simulink model "GFOL_nonlinear"  (R2020a)
settings: Solver=ode3  StartTime=0.0  StopTime=Tsim  FixedStep=T_solver  RelTol=1e-6
values from neighbouring files (symbols this model uses):
  f_n1 = f1    (= 50)    [param.m]
  Ipeak_n1 = Sn_n1*sqrt(2)/(sqrt(3)*Un_n1)    [linearization_point.m]    (also in param.m = Sn_n1/(sqrt(3)*Un_n1))
  k_droop_f_n1 = 20*Sn_n1/w_n1    (= 175070.437401)    [param.m]
  k_droop_u_n1 = 0.3*50*Sn_n1/Vpeak_n1    [param.m]
  ki_P_n1 = 1e-3*1/tau_p    (= 0.01)    [param.m]
  ki_pll_n1 = kp_pll_n1/tau_pll_n1    [param.m]
  ki_Q_n1 = 1e-3*1/tau_q    (= 0.01)    [param.m]
  ki_s_n1 = Rc_n1/taus    (= 0.865636363636)    [param.m]
  kp_P_n1 = 1e-3*taus/tau_p    (= 1e-05)    [param.m]
  kp_pll_n1 = xi_pll_n1*2*omega_pll_n1/Vpeak_n1    [param.m]
  kp_Q_n1 = 1e-3*taus/tau_q    (= 1e-05)    [param.m]
  kp_s_n1 = Lc_n1/taus    (= 0.0826621837157)    [param.m]
  Lc_n1 = 0.15*Ln_n1    (= 8.26621837157e-05)    [param.m]
  Lg_n1 = Xg_n1/w_g1    [param.m]
  Lg_n2 = imag(Zg_n2)/w_g1    [param.m]
  P_ref_n1 = 0.5*Sn_n1    (= 1375000)    [param.m]
  plots_step = 10e-6    (= 1e-05)    [param.m]
  Q_ref_n1 = 0.1*Sn_n1    (= 275000)    [param.m]
  Rc_n1 = 0.005*Xn_n1    (= 0.000865636363636)    [param.m]
  Rg_n1 = sqrt(Xcc1^2/(XR_ratio^2+1))    [param.m]
  Rg_n2 = real(Zg_n2)    [param.m]
  Sn_n1 = Sn1    (= 2750000)    [param.m]
  T_solver = 10e-6    (= 1e-05)    [param.m]
  T_step = 2    [param.m]
  tau_droop_f = 1/50    (= 0.02)    [param.m]
  tau_droop_u = 1/50    (= 0.02)    [param.m]
  Vdcref_n1 = 2e3    (= 2000)    [param.m]
  Vpeak_g1_fnl = Vpeak_n1*0.98    [param.m]
  Vpeak_n1 = Un_n1/sqrt(3)*sqrt(2)    [param.m]
  Vpeak_q1_init = Vpeak_n1*1    [param.m]
  w_n1 = 2*pi*f_n1    (= 314.159265359)    [param.m]
undefined symbols (not defined in the file or in its folder): P_set, P_step, Q_set, Q_step, t_ramp, t_step_P, t_step_Q, tau_ramp
libraries: powerlib x37, simulink x5, simulink_extras x1
(part 1 of 2)
settings Model: SimulationMode=accelerator  ExtModeTrigDuration=100  Creator=Enric  LastModifiedBy=Saman
settings SolverCC: SolverJacobianMethodControl=FullPerturbation  AutoInsertRateTranBlk=on
settings DataIOCC: LimitDataPoints=on  SaveOutput=off  ReturnWorkspaceOutputs=off  StateSaveName=tmp_raccel_xout  SignalLoggingName=tmp_raccel_logsout
settings OptimizationCC: EfficientMapNaN2IntZero=off  LifeSpan=inf
settings DebuggingCC: AllowSymbolicDim=off  SFUnexpectedBacktrackingDiag=warning  SFNoUnconditionalDefaultTransitionDiag=warning  SFExecutionAtInitializationDiag=none  ArithmeticOperatorsInVariantConditions=warning
settings HardwareCC: TargetBitPerPointer=64  TargetBitPerSizeT=64  TargetBitPerPtrDiffT=64  TargetLongLongMode=on  TargetIntDivRoundTo=Zero  TargetEndianess=LittleEndian  TargetWordSize=64  TargetHWDeviceType=MATLAB Host  ProdEqTarget=off
settings ModelReferenceCC: PropagateSignalLabelsOutOfModel=off
settings SFSimCC: SimUseLocalCustomCode=off  CustomCodeUndefinedFunction=UseInterfaceOnly
settings RTWCC: SystemTargetFile=raccel.tlc  TemplateMakefile=raccel_default_tmf  RTWVerbose=off  RTWUseLocalCustomCode=off  RTWUseSimCustomCode=on
settings CodeAppCC: GenerateComments=off  MaxIdLength=128  MangleLength=10  SimulinkBlockComments=off
settings RaccelTargetCC: MultiInstanceERTCode=off  ENABLE_SLEXEC_SSBRIDGE=0  RTWCAPISignals=off  RTWCAPIParams=on  RTWCAPIRootIO=off
settings ConfigComp: CovMetricSettings=dw  CovHtmlReporting=on  CovSaveCumulativeToWorkspaceVar=on  CovSaveSingleToWorkspaceVar=on  CovExternalEMLEnable=off
settings SimscapeCC: SimscapeNormalizeSystem=off

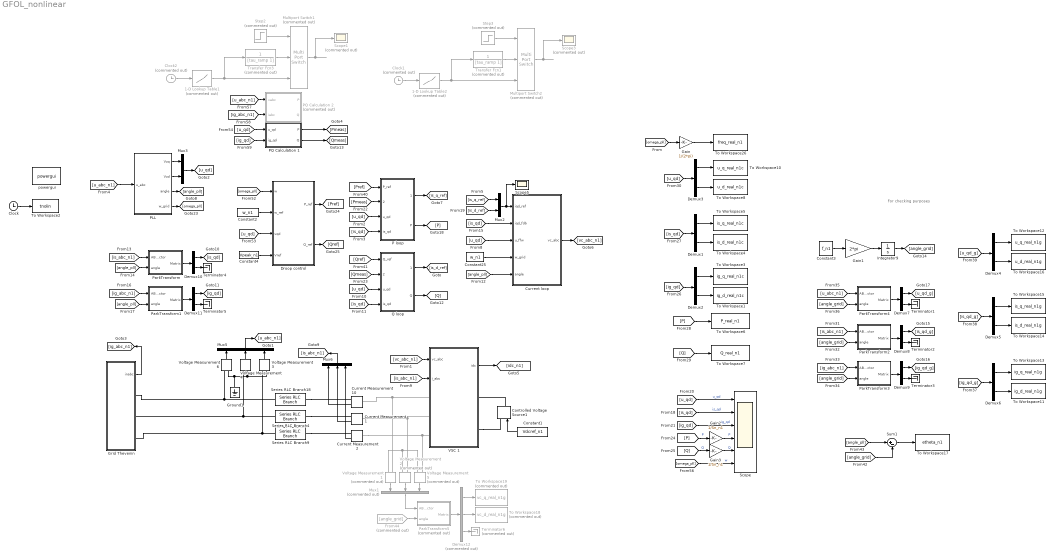
== system GFOL_nonlinear ==
  note: For checking purposes
  1-D Lookup Table1 : Lookup_n-D  Commented=on  NumberOfTableDimensions=1  BreakpointsForDimension1=[0,t_ramp,t_step_P]  Table=[0,P_set,P_step]  InterpMethod=Flat  InternalRulePriority=Speed  RndMeth=Simplest  InputSameDT=on
  1-D Lookup Table2 : Lookup_n-D  Commented=on  NumberOfTableDimensions=1  BreakpointsForDimension1=[0,t_ramp,t_step_Q]  Table=[0,Q_set,Q_step]  InterpMethod=Flat  InternalRulePriority=Speed  RndMeth=Simplest  InputSameDT=on
  Clock : Clock
  Clock1 : Clock  Commented=on
  Clock2 : Clock  Commented=on
  Constant1 : Constant  Value=Vdcref_n1
  Constant2 : Constant  Value=w_n1
  Constant25 : Constant  Value=w_n1
  Constant3 : Constant  Value=f_n1
  Constant4 : Constant  Value=Vpeak_n1
  Controlled Voltage Source1 : powerlib/Electrical Sources/Controlled Voltage Source  Initialize=off  Source_Type=DC  Amplitude=Vdcref_n1  Phase=0  Frequency=0  Measurements=None
  Current Measurement1 : powerlib/Measurements/Current Measurement  PhasorSimulation=off  OutputType=Complex  PSBequivalent=0
  Current Measurement10 : powerlib/Measurements/Current Measurement  PhasorSimulation=off  OutputType=Complex  PSBequivalent=0
  Current Measurement2 : powerlib/Measurements/Current Measurement  PhasorSimulation=off  OutputType=Complex  PSBequivalent=0
  Current loop : Subsystem
  Demux{1..11} (11 alike) : Demux  Outputs=2
  Demux12 : Demux  Commented=on  Outputs=3
  Droop control : Subsystem
  From44 : From  Commented=on  GotoTag=angle_grid
  Gain : Gain  Gain=1/(2*pi)
  Gain1 : Gain  Gain=2*pi
  Gain2 : Gain  Gain=1/Sn_n1
  Gain3 : Gain  Gain=1/Sn_n1
  Grid Thevenin : Subsystem
  Ground1 : powerlib/Elements/Ground  LConnTagsString=a
  Integrator9 : Integrator
  Multiport Switch1 : MultiPortSwitch  Commented=on  Inputs=2
  Multiport Switch2 : MultiPortSwitch  Commented=on  Inputs=2
  Mux1 : Mux  Commented=on  Inputs=3
  Mux2 : Mux  Inputs=2
  Mux3 : Mux  Inputs=2
  Mux5 : Mux  Inputs=3
  Mux6 : Mux  Inputs=3
  P loop : Subsystem
  PLL : Subsystem
  PQ Calculation 1 : Subsystem
  PQ Calculation 2 : Subsystem  Commented=on
  ParkTransform : Subsystem  mask(Gerard){}
      mask help:
      | This block applies the park transfomation from a desired vector.
      | The input Xabc refers to the vector in the ABC frame, and the second input is the angle used in the transformation.
      | The output is the vector in the qd0 frame.
      mask Display:
      | port_label('output',1,'Xqd0')
      | port_label('input',1,'Xabc')
      | port_label('input',2,'angle')
  ParkTransform1 : Subsystem  mask(Gerard){}
      mask help:
      | This block applies the park transfomation from a desired vector.
      | The input Xabc refers to the vector in the ABC frame, and the second input is the angle used in the transformation.
      | The output is the vector in the qd0 frame.
      mask Display:
      | port_label('output',1,'Xqd0')
      | port_label('input',1,'Xabc')
      | port_label('input',2,'angle')
  ParkTransform2 : Subsystem  mask(Gerard){}
      mask help:
      | This block applies the park transfomation from a desired vector.
      | The input Xabc refers to the vector in the ABC frame, and the second input is the angle used in the transformation.
      | The output is the vector in the qd0 frame.
      mask Display:
      | port_label('output',1,'Xqd0')
      | port_label('input',1,'Xabc')
      | port_label('input',2,'angle')
  ParkTransform3 : Subsystem  mask(Gerard){}
      mask help:
      | This block applies the park transfomation from a desired vector.
      | The input Xabc refers to the vector in the ABC frame, and the second input is the angle used in the transformation.
      | The output is the vector in the qd0 frame.
      mask Display:
      | port_label('output',1,'Xqd0')
      | port_label('input',1,'Xabc')
      | port_label('input',2,'angle')
  ParkTransform4 : Subsystem  mask(Gerard){}
      mask help:
      | This block applies the park transfomation from a desired vector.
      | The input Xabc refers to the vector in the ABC frame, and the second input is the angle used in the transformation.
      | The output is the vector in the qd0 frame.
      mask Display:
      | port_label('output',1,'Xqd0')
      | port_label('input',1,'Xabc')
      | port_label('input',2,'angle')
  ParkTransform5 : Subsystem  Commented=on  mask(Gerard){}
      mask help:
      | This block applies the park transfomation from a desired vector.
      | The input Xabc refers to the vector in the ABC frame, and the second input is the angle used in the transformation.
      | The output is the vector in the qd0 frame.
      mask Display:
      | port_label('output',1,'Xqd0')
      | port_label('input',1,'Xabc')
      | port_label('input',2,'angle')
  Q loop : Subsystem
  Scope : Scope  NumInputPorts=6
  Scope1 : Scope  Commented=on
  Scope3 : Scope  Commented=on
  Scope5 : Scope
  Series RLC Branch18 : powerlib/Elements/Series RLC Branch  LConnTagsString=__new0  RConnTagsString=__new0  BranchType=RL  Resistance=Rc_n1  Inductance=Lc_n1  SetiL0=off  InitialCurrent=10  Capacitance=0  Setx0=off  InitialVoltage=0  Measurements=None
  Series RLC Branch4 : powerlib/Elements/Series RLC Branch  LConnTagsString=__new0  RConnTagsString=__new0  BranchType=RL  Resistance=Rc_n1  Inductance=Lc_n1  SetiL0=off  InitialCurrent=10  Capacitance=0  Setx0=off  InitialVoltage=0  Measurements=None
  Series RLC Branch9 : powerlib/Elements/Series RLC Branch  LConnTagsString=__new0  RConnTagsString=__new0  BranchType=RL  Resistance=Rc_n1  Inductance=Lc_n1  SetiL0=off  InitialCurrent=10  Capacitance=0  Setx0=off  InitialVoltage=0  Measurements=None
  Step2 : Step  Commented=on  Time=t_step_P-0.01  Before=1  After=2  SampleTime=0
  Step3 : Step  Commented=on  Time=t_step_Q-0.01  Before=1  After=2  SampleTime=0
  Sum1 : Sum  Inputs=|+-
  Terminator{1..5} (5 alike) : Terminator
  Terminator6 : Terminator  Commented=on
  To Workspace1 : ToWorkspace  VariableName=ig_d_real_n1c  SampleTime=plots_step
  To Workspace10 : ToWorkspace  VariableName=u_q_real_n1c  SampleTime=plots_step
  To Workspace11 : ToWorkspace  VariableName=ig_d_real_n1g  SampleTime=plots_step
  To Workspace12 : ToWorkspace  VariableName=u_q_real_n1g  SampleTime=plots_step
  To Workspace13 : ToWorkspace  VariableName=ig_q_real_n1g  SampleTime=plots_step
  To Workspace14 : ToWorkspace  VariableName=is_d_real_n1g  SampleTime=plots_step
  To Workspace15 : ToWorkspace  VariableName=is_q_real_n1g  SampleTime=plots_step
  To Workspace16 : ToWorkspace  VariableName=u_d_real_n1g  SampleTime=plots_step
  To Workspace17 : ToWorkspace  VariableName=etheta_n1  SampleTime=plots_step
  To Workspace18 : ToWorkspace  Commented=on  VariableName=vc_d_real_n1g  SampleTime=plots_step
  To Workspace19 : ToWorkspace  Commented=on  VariableName=vc_q_real_n1g  SampleTime=plots_step
  To Workspace2 : ToWorkspace  VariableName=tnolin  SampleTime=plots_step
  To Workspace26 : ToWorkspace  VariableName=freq_real_n1  SampleTime=plots_step
  To Workspace3 : ToWorkspace  VariableName=ig_q_real_n1c  SampleTime=plots_step
  To Workspace4 : ToWorkspace  VariableName=is_d_real_n1c  SampleTime=plots_step
  To Workspace5 : ToWorkspace  VariableName=is_q_real_n1c  SampleTime=plots_step
  To Workspace6 : ToWorkspace  VariableName=P_real_n1  SampleTime=plots_step
  To Workspace7 : ToWorkspace  VariableName=Q_real_n1  SampleTime=plots_step
  To Workspace8 : ToWorkspace  VariableName=u_d_real_n1c  SampleTime=plots_step
  Transfer Fcn1 : TransferFcn  Commented=on  Denominator=[tau_ramp 1]
  Transfer Fcn3 : TransferFcn  Commented=on  Denominator=[tau_ramp 1]
  VSC 1 : Subsystem
  Voltage Measurement1 : powerlib/Measurements/Voltage Measurement  Commented=on  PhasorSimulation=off  OutputType=Complex  PSBequivalent=0
  Voltage Measurement2 : powerlib/Measurements/Voltage Measurement  Commented=on  PhasorSimulation=off  OutputType=Complex  PSBequivalent=0
  Voltage Measurement3 : powerlib/Measurements/Voltage Measurement  PhasorSimulation=off  OutputType=Complex  PSBequivalent=0
  Voltage Measurement4 : powerlib/Measurements/Voltage Measurement  PhasorSimulation=off  OutputType=Complex  PSBequivalent=0
  Voltage Measurement5 : powerlib/Measurements/Voltage Measurement  Commented=on  PhasorSimulation=off  OutputType=Complex  PSBequivalent=0
  Voltage Measurement6 : powerlib/Measurements/Voltage Measurement  PhasorSimulation=off  OutputType=Complex  PSBequivalent=0
  powergui : powerlib/powergui  Priority=1  SimulationMode=Continuous  SampleTime=T_solver  frequency=60  Iterations=50  frequencyindice=0  Pbase=100e6  ErrMax=1e-4  UnitsV=kV  UnitsW=MW  buscounter=0  FunctionMessages=off  echomessages=off  EnableUseOfTLC=off  CurrentSourceSwitches=off  DisableSnubberDevices=off  DisableRonSwitches=off  DisableVfSwitches=off  DisplayEquations=off  AutomaticDiscreteSolvers=off  SolverType=Tustin  Interpol=off  ExternalGateDelay=off  methode=off  Ts=0  x0status=blocks  SPID=off  SwTol=0  HookPort=off  NonlinearTolerance=1e-4  nMaxIteration=100  ContinueOnMaxIteration=off  RestoreLinks=warning  ResistiveCurrentMeasurement=off  Frange=[0:2:500]  Ylog=off  Xlog=on  ShowGrid=off  save=off  variable=ZData  structure=Vk  ZoomFFT=off  StartTime=2.01  cycles=3  DisplayStyle=1  fundamental=50  FreqAxis=off  MaxFrequency=1000  frequencyindicesteady=1  RmsSteady=1  display=off
  wires:
  Voltage Measurement4/1 -> Mux5/2
  Voltage Measurement3/1 -> Mux5/3
  Voltage Measurement6/1 -> Mux5/1
  Clock/1 -> To Workspace2/1
  Mux5/1 -> [u_abc_n1]
  Grid Thevenin/1(inabc) -> [ig_abc_n1]
  VSC 1/1(idc) -> [idc_n1]
  Voltage Measurement1/1 -> Mux1/1
  Voltage Measurement2/1 -> Mux1/2
  Voltage Measurement5/1 -> Mux1/3
  Constant1/1 -> Controlled Voltage Source1/1
  [u_qd] -> Current loop/3(u_ffw)
  Constant25/1 -> Current loop/4(w_grid)
  Mux2/1 -> Scope5/1, Current loop/1(iqd_ref)
  [is_qd] -> Current loop/2(iqd_fdb)
  Mux1/1 -> ParkTransform5/1(ABC vector)
  PLL/4(w_grid) -> [omega_pll]
  PLL/1(Vzq) -> Mux3/1
  PLL/2(Vzd) -> Mux3/2
  PLL/3(angle) -> [angle_pll]
  [is_abc_n1] -> VSC 1/2(i_abc)
  Current loop/1(vc_abc) -> [vc_abc_n1]
  [vc_abc_n1] -> VSC 1/1(vc_abc)
  [u_qd] -> P loop/3(u_qd)
  [is_qd] -> P loop/4(is_qd)
  [u_qd] -> Q loop/3(u_qd)
  [is_qd] -> Q loop/4(is_qd)
  [angle_pll] -> Current loop/5(angle)
  Current Measurement1/1 -> Mux6/2
  Current Measurement2/1 -> Mux6/3
  Current Measurement10/1 -> Mux6/1
  Mux6/1 -> [is_abc_n1]
  [angle_pll] -> ParkTransform/2(angle)
  [is_abc_n1] -> ParkTransform/1(ABC vector)
  [angle_pll] -> ParkTransform1/2(angle)
  [ig_abc_n1] -> ParkTransform1/1(ABC vector)
  ParkTransform1/1(Matrix) -> Demux11/1
  [u_qd] -> Scope/1  "u_qd"
  [is_qd] -> Scope/2  "is_qd"
  [ig_qd] -> Scope/3  "ig_qd"
  P loop/2(P) -> [P]
  Q loop/2(Q) -> [Q]
  Gain2/1 -> Scope/4  "P"
  Gain3/1 -> Scope/5  "Q"
  [P] -> To Workspace6/1
  [Q] -> To Workspace7/1
  Demux3/2 -> To Workspace8/1
  Demux3/1 -> To Workspace10/1
  [u_qd] -> Demux3/1
  Constant3/1 -> Gain1/1
  Gain1/1 -> Integrator9/1
  Integrator9/1 -> [angle_grid]
  [ig_abc_n1] -> ParkTransform3/1(ABC vector)
  [angle_grid] -> ParkTransform3/2(angle)
  [is_abc_n1] -> ParkTransform2/1(ABC vector)
  [angle_grid] -> ParkTransform2/2(angle)
  [angle_grid] -> ParkTransform4/2(angle)
  [u_abc_n1] -> ParkTransform4/1(ABC vector)
  ParkTransform4/1(Matrix) -> Demux7/1
  Transfer Fcn3/1 -> Multiport Switch1/2
  1-D Lookup Table1/1 -> Multiport Switch1/3, Transfer Fcn3/1
  Clock2/1 -> 1-D Lookup Table1/1
  Step2/1 -> Multiport Switch1/1
  Multiport Switch1/1 -> Scope1/1
  [Pref] -> P loop/1(P_ref)
  Multiport Switch2/1 -> Scope3/1
  Step3/1 -> Multiport Switch2/1
  Clock1/1 -> 1-D Lookup Table2/1
  1-D Lookup Table2/1 -> Transfer Fcn1/1, Multiport Switch2/3
  Transfer Fcn1/1 -> Multiport Switch2/2
  [Qref] -> Q loop/1(Q_ref)
  [is_qd] -> Demux1/1
  Demux1/1 -> To Workspace5/1
  Demux1/2 -> To Workspace4/1
  Demux2/2 -> To Workspace1/1
  Demux2/1 -> To Workspace3/1
  [ig_qd] -> Demux2/1
  Demux4/1 -> To Workspace12/1
  [u_qd_g] -> Demux4/1
  Demux4/2 -> To Workspace16/1
  Demux5/2 -> To Workspace14/1
  [is_qd_g] -> Demux5/1
  Demux5/1 -> To Workspace15/1
  [ig_qd_g] -> Demux6/1
  Demux6/1 -> To Workspace13/1
  Demux6/2 -> To Workspace11/1
  Demux7/1 -> [u_qd_g]
  Demux8/1 -> [is_qd_g]
  ParkTransform2/1(Matrix) -> Demux8/1
  Demux9/1 -> [ig_qd_g]
  ParkTransform3/1(Matrix) -> Demux9/1
  Demux7/2 -> Terminator1/1
  Demux8/2 -> Terminator2/1
  Demux9/2 -> Terminator3/1
  ParkTransform/1(Matrix) -> Demux10/1
  Demux10/1 -> [is_qd]
  Demux10/2 -> Terminator4/1
  Demux11/2 -> Terminator5/1
  Demux11/1 -> [ig_qd]
  [angle_pll] -> Sum1/1
  [angle_grid] -> Sum1/2
  Sum1/1 -> To Workspace17/1
  [is_q_ref] -> Mux2/1
  [is_d_ref] -> Mux2/2
  ParkTransform5/1(Matrix) -> Demux12/1
  Demux12/2 -> To Workspace18/1
  From44/1 -> ParkTransform5/2(angle)
  Demux12/1 -> To Workspace19/1
  Demux12/3 -> Terminator6/1
  [omega_pll] -> Droop control/1(w)
  Constant2/1 -> Droop control/2(w_ref)
  Droop control/1(P_ref) -> [Pref]
  Droop control/2(Q_ref) -> [Qref]
  [u_qd] -> Droop control/3(vqd)
  Constant4/1 -> Droop control/4(Vref)
  [u_qd] -> PQ Calculation 1/1(u_qd)
  [ig_qd] -> PQ Calculation 1/2(ig_qd)
  [u_abc_n1] -> PLL/1(u_abc)
  Mux3/1 -> [u_qd]
  Gain/1 -> To Workspace26/1
  [omega_pll] -> Gain/1
  [Pmeas] -> P loop/2(P_meas)
  [Qmeas] -> Q loop/2(Q_meas)
  P loop/1(is_q_ref) -> [is_q_ref]
  Q loop/1(is_d_ref) -> [is_d_ref]
  [omega_pll] -> Scope/6  "w"
  [u_abc_n1] -> PQ Calculation 2/1(vabc)
  [ig_abc_n1] -> PQ Calculation 2/2(iabc)
  PQ Calculation 1/2(Q) -> [Qmeas]
  PQ Calculation 1/1(P) -> [Pmeas]
  [P] -> Gain2/1  "P"
  [Q] -> Gain3/1  "Q"
  connections:
  Voltage Measurement5/LConn1 -- Current Measurement2/LConn1 -- VSC 1/LConn3
  Voltage Measurement1/LConn1 -- VSC 1/LConn1 -- Current Measurement10/LConn1
  Voltage Measurement2/LConn1 -- Current Measurement1/LConn1 -- VSC 1/LConn2
  Controlled Voltage Source1/RConn1 -- VSC 1/RConn1
  VSC 1/RConn2 -- Controlled Voltage Source1/LConn1
  Grid Thevenin/RConn1 -- Voltage Measurement6/LConn1 -- Series RLC Branch18/LConn1
  Voltage Measurement1/LConn2 -- Voltage Measurement2/LConn2 -- Voltage Measurement5/LConn2
  Series RLC Branch18/RConn1 -- Current Measurement10/RConn1
  Series RLC Branch4/RConn1 -- Current Measurement1/RConn1
  Series RLC Branch9/RConn1 -- Current Measurement2/RConn1
  Grid Thevenin/RConn3 -- Series RLC Branch9/LConn1 -- Voltage Measurement3/LConn1
  Grid Thevenin/RConn2 -- Series RLC Branch4/LConn1 -- Voltage Measurement4/LConn1
  Voltage Measurement6/LConn2 -- Ground1/LConn1 -- Voltage Measurement3/LConn2 -- Voltage Measurement4/LConn2

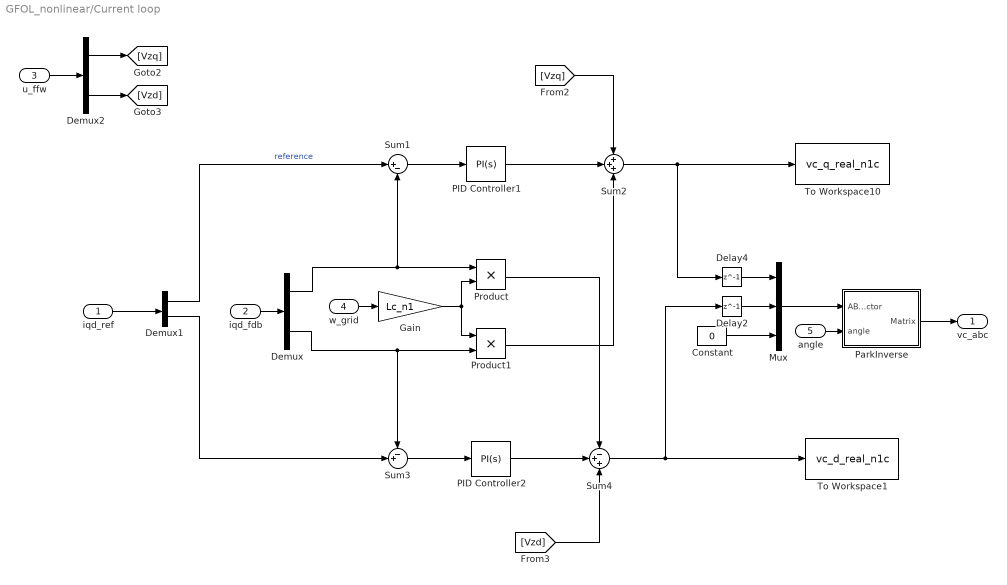
== system GFOL_nonlinear/Current loop ==
  iqd_ref : Inport
  iqd_fdb : Inport  Port=2
  u_ffw : Inport  Port=3
  w_grid : Inport  Port=4
  angle : Inport  Port=5
  Constant : Constant  Value=0
  Delay2 : Delay  DelayLength=1  InitialCondition=0  SampleTime=T_solver
  Delay4 : Delay  DelayLength=1  InitialCondition=Vpeak_n1  SampleTime=T_solver
  Demux : Demux  Outputs=2
  Demux1 : Demux  Outputs=2
  Demux2 : Demux  Outputs=2
  Gain : Gain  Gain=Lc_n1
  Mux : Mux  Inputs=3
  PID Controller1 : simulink/Continuous/PID Controller  Controller=PI  Form=Parallel  TimeDomain=Continuous-time  UseExternalTs=off  SampleTime=-1  IntegratorMethod=Forward Euler  FilterMethod=Forward Euler  ControllerParametersSource=internal  P=kp_s_n1  I=ki_s_n1  D=0  UseFilter=on  N=100  TunerSelectOption=Transfer Function Based (PID Tuner App)  InitialConditionSource=internal  InitialConditionForIntegrator=0  InitialConditionForFilter=0  DifferentiatorICPrevScaledInput=0  ExternalReset=none  TrackingMode=off  Kt=1  LimitOutput=off  UpperSaturationLimit=inf  LowerSaturationLimit=-inf  LinearizeAsGain=on  AntiWindupMode=none  Kb=1  POutMin=[]  POutMax=[]  IOutMin=[]  IOutMax=[]  DOutMin=[]  DOutMax=[]  NOutMin=[]  NOutMax=[]  SumOutMin=[]  SumOutMax=[]  SaturationOutMin=[]  SaturationOutMax=[]  PParamMin=[]  PParamMax=[]  IParamMin=[]  IParamMax=[]  DParamMin=[]  DParamMax=[]  NParamMin=[]  NParamMax=[]  KbParamMin=[]  KbParamMax=[]  KtParamMin=[]  KtParamMax=[]  KbOutMin=[]  KbOutMax=[]  KtOutMin=[]  KtOutMax=[]  IntegratorOutMin=[]  IntegratorOutMax=[]  FilterOutMin=[]  FilterOutMax=[]  SumI1OutMin=[]  SumI1OutMax=[]  SumI2OutMin=[]  SumI2OutMax=[]  SumI3OutMin=[]  SumI3OutMax=[]  SumI4OutMin=[]  SumI4OutMax=[]  SumDOutMin=[]  SumDOutMax=[]  DifferentiatorOutMin=[]  DifferentiatorOutMax=[]  FilterDiffOutCoefMin=[]  FilterDiffOutCoefMax=[]  ReciprocalOutMin=[]  ReciprocalOutMax=[]  SumDenOutMin=[]  SumDenOutMax=[]  SumNumOutMin=[]  SumNumOutMax=[]  DivideOutMin=[]  DivideOutMax=[]  UdiffTsProdOutMin=[]  UdiffTsProdOutMax=[]  NTsProdOutMin=[]  NTsProdOutMax=[]  UintegralTsProdOutMin=[]  UintegralTsProdOutMax=[]  UngainTsProdOutMin=[]  UngainTsProdOutMax=[]  IntegratorContinuousStateAttributes=''  IntegratorStateMustResolveToSignalObject=off  IntegratorRTWStateStorageClass=Auto  FilterContinuousStateAttributes=''  FilterStateMustResolveToSignalObject=off  FilterRTWStateStorageClass=Auto  ParallelPVariant=InternalParameters  IdealPVariant=Disabled  IVariant=InternalParameters  DVariant=Disabled  IntegratorVariant=Continuous  SatVariant=Disabled  AWVariant=Passthrough  PCopyVariant=Disabled  TRVariant=Disabled  FdbkBlocksVariant=Forward  IdealPFdbkVariant=Disabled  SatFdbkVariant=Disabled  DerivativeFilterVariant=Disabled  NVariant=Disabled  NCopyVariant=Disabled_SignalSpec  FilterICVariant=Disabled  IntegratorICVariant=InternalICs  ExternalResetVariant=Disabled  TRSumVariant=Passthrough  SumFdbkVariant=Disabled  SumVariant=Sum_PI  TsampFilterVariant=InternalTs  TsampNgainVariant=Passthrough  TsampIntegralVariant=Passthrough
  PID Controller2 : simulink/Continuous/PID Controller  Controller=PI  Form=Parallel  TimeDomain=Continuous-time  UseExternalTs=off  SampleTime=-1  IntegratorMethod=Forward Euler  FilterMethod=Forward Euler  ControllerParametersSource=internal  P=kp_s_n1  I=ki_s_n1  D=0  UseFilter=on  N=100  TunerSelectOption=Transfer Function Based (PID Tuner App)  InitialConditionSource=internal  InitialConditionForIntegrator=0  InitialConditionForFilter=0  DifferentiatorICPrevScaledInput=0  ExternalReset=none  TrackingMode=off  Kt=1  LimitOutput=off  UpperSaturationLimit=inf  LowerSaturationLimit=-inf  LinearizeAsGain=on  AntiWindupMode=none  Kb=1  POutMin=[]  POutMax=[]  IOutMin=[]  IOutMax=[]  DOutMin=[]  DOutMax=[]  NOutMin=[]  NOutMax=[]  SumOutMin=[]  SumOutMax=[]  SaturationOutMin=[]  SaturationOutMax=[]  PParamMin=[]  PParamMax=[]  IParamMin=[]  IParamMax=[]  DParamMin=[]  DParamMax=[]  NParamMin=[]  NParamMax=[]  KbParamMin=[]  KbParamMax=[]  KtParamMin=[]  KtParamMax=[]  KbOutMin=[]  KbOutMax=[]  KtOutMin=[]  KtOutMax=[]  IntegratorOutMin=[]  IntegratorOutMax=[]  FilterOutMin=[]  FilterOutMax=[]  SumI1OutMin=[]  SumI1OutMax=[]  SumI2OutMin=[]  SumI2OutMax=[]  SumI3OutMin=[]  SumI3OutMax=[]  SumI4OutMin=[]  SumI4OutMax=[]  SumDOutMin=[]  SumDOutMax=[]  DifferentiatorOutMin=[]  DifferentiatorOutMax=[]  FilterDiffOutCoefMin=[]  FilterDiffOutCoefMax=[]  ReciprocalOutMin=[]  ReciprocalOutMax=[]  SumDenOutMin=[]  SumDenOutMax=[]  SumNumOutMin=[]  SumNumOutMax=[]  DivideOutMin=[]  DivideOutMax=[]  UdiffTsProdOutMin=[]  UdiffTsProdOutMax=[]  NTsProdOutMin=[]  NTsProdOutMax=[]  UintegralTsProdOutMin=[]  UintegralTsProdOutMax=[]  UngainTsProdOutMin=[]  UngainTsProdOutMax=[]  IntegratorContinuousStateAttributes=''  IntegratorStateMustResolveToSignalObject=off  IntegratorRTWStateStorageClass=Auto  FilterContinuousStateAttributes=''  FilterStateMustResolveToSignalObject=off  FilterRTWStateStorageClass=Auto  ParallelPVariant=InternalParameters  IdealPVariant=Disabled  IVariant=InternalParameters  DVariant=Disabled  IntegratorVariant=Continuous  SatVariant=Disabled  AWVariant=Passthrough  PCopyVariant=Disabled  TRVariant=Disabled  FdbkBlocksVariant=Forward  IdealPFdbkVariant=Disabled  SatFdbkVariant=Disabled  DerivativeFilterVariant=Disabled  NVariant=Disabled  NCopyVariant=Disabled_SignalSpec  FilterICVariant=Disabled  IntegratorICVariant=InternalICs  ExternalResetVariant=Disabled  TRSumVariant=Passthrough  SumFdbkVariant=Disabled  SumVariant=Sum_PI  TsampFilterVariant=InternalTs  TsampNgainVariant=Passthrough  TsampIntegralVariant=Passthrough
  ParkInverse : Subsystem  mask(Gerard){}
      mask help:
      | This block applies the park inverse transfomation from a desired vector.
      | The input Xqd0 refers to the vector in the qd0 frame, and the second input is the angle used in the inverse transformation.
      | The output is the vector in the ABC frame.
      mask Display:
      | port_label('output',1,'Xabc')
      | port_label('input',1,'Xqd0')
      | port_label('input',2,'angle')
  Product : Product  RndMeth=Zero
  Product1 : Product  RndMeth=Zero
  Sum1 : Sum  Inputs=|+-
  Sum2 : Sum  Inputs=+++
  Sum3 : Sum  Inputs=-+|
  Sum4 : Sum  Inputs=-++
  To Workspace1 : ToWorkspace  VariableName=vc_d_real_n1c  SampleTime=plots_step
  To Workspace10 : ToWorkspace  VariableName=vc_q_real_n1c  SampleTime=plots_step
  vc_abc : Outport
  wires:
  iqd_fdb/1 -> Demux/1
  w_grid/1 -> Gain/1
  PID Controller1/1 -> Sum2/2
  Demux/1 -> Sum1/2, Product/1
  Gain/1 -> Product1/1, Product/2
  Demux/2 -> Product1/2, Sum3/1
  Product1/1 -> Sum2/3
  Product/1 -> Sum4/1
  Constant/1 -> Mux/3
  ParkInverse/1(Matrix) -> vc_abc/1
  [Vzq] -> Sum2/1
  Mux/1 -> ParkInverse/1(ABC vector)
  Demux2/1 -> [Vzq]
  Demux2/2 -> [Vzd]
  u_ffw/1 -> Demux2/1
  [Vzd] -> Sum4/3
  angle/1 -> ParkInverse/2(angle)
  Sum1/1 -> PID Controller1/1
  Sum3/1 -> PID Controller2/1
  PID Controller2/1 -> Sum4/2
  Demux1/2 -> Sum3/2
  Demux1/1 -> Sum1/1  "reference"
  iqd_ref/1 -> Demux1/1
  Sum4/1 -> Delay2/1, To Workspace1/1
  Sum2/1 -> To Workspace10/1, Delay4/1
  Delay2/1 -> Mux/2
  Delay4/1 -> Mux/1

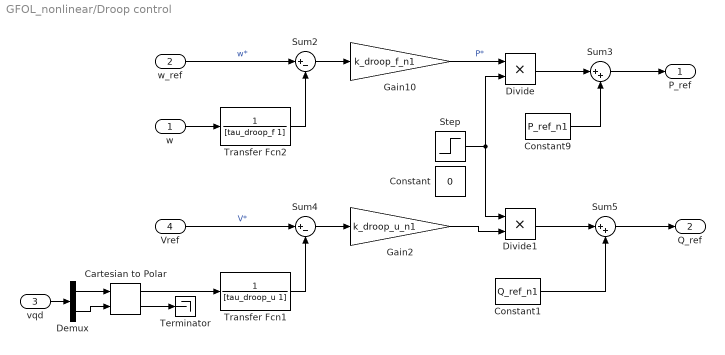
== system GFOL_nonlinear/Droop control ==
  w : Inport
  w_ref : Inport  Port=2
  vqd : Inport  Port=3
  Vref : Inport  Port=4
  Cartesian to Polar : simulink_extras/Transformations/Cartesian to Polar
  Constant : Constant  Value=0
  Constant1 : Constant  Value=Q_ref_n1
  Constant9 : Constant  Value=P_ref_n1
  Demux : Demux  Outputs=2
  Divide : Product  Inputs=**
  Divide1 : Product  Inputs=**
  Gain10 : Gain  Gain=k_droop_f_n1
  Gain2 : Gain  Gain=k_droop_u_n1
  Step : Step  Time=0.5  SampleTime=0
  Sum2 : Sum  Inputs=|+-
  Sum3 : Sum  Inputs=|++
  Sum4 : Sum  Inputs=|+-
  Sum5 : Sum  Inputs=|++
  Terminator : Terminator
  Transfer Fcn1 : TransferFcn  Denominator=[tau_droop_u 1]
  Transfer Fcn2 : TransferFcn  Denominator=[tau_droop_f 1]
  P_ref : Outport
  Q_ref : Outport  Port=2
  wires:
  w_ref/1 -> Sum2/1  "w*"
  Sum2/1 -> Gain10/1
  w/1 -> Transfer Fcn2/1
  Transfer Fcn2/1 -> Sum2/2
  Transfer Fcn1/1 -> Sum4/2
  Vref/1 -> Sum4/1  "V*"
  Sum4/1 -> Gain2/1
  Constant1/1 -> Sum5/2
  Gain10/1 -> Divide/1  "P*"
  vqd/1 -> Demux/1
  Demux/1 -> Cartesian to Polar/1
  Demux/2 -> Cartesian to Polar/2
  Cartesian to Polar/2 -> Terminator/1
  Cartesian to Polar/1 -> Transfer Fcn1/1
  Constant9/1 -> Sum3/2
  Gain2/1 -> Divide1/2
  Divide/1 -> Sum3/1
  Step/1 -> Divide1/1, Divide/2
  Divide1/1 -> Sum5/1
  Sum3/1 -> P_ref/1
  Sum5/1 -> Q_ref/1

== system GFOL_nonlinear/Grid Thevenin ==
  note: Grid Thevenin
  Controlled Voltage Source3 : powerlib/Electrical Sources/Controlled Voltage Source  Initialize=off  Source_Type=AC  Amplitude=Vpeak_n1  Phase=0  Frequency=50  Measurements=None
  Controlled Voltage Source4 : powerlib/Electrical Sources/Controlled Voltage Source  Initialize=off  Source_Type=AC  Amplitude=Vpeak_n1  Phase=-120  Frequency=50  Measurements=None
  Controlled Voltage Source5 : powerlib/Electrical Sources/Controlled Voltage Source  Initialize=off  Source_Type=AC  Amplitude=Vpeak_n1  Phase=120  Frequency=50  Measurements=None
  Current Measurement1 : powerlib/Measurements/Current Measurement  PhasorSimulation=off  OutputType=Complex  PSBequivalent=0
  Current Measurement10 : powerlib/Measurements/Current Measurement  PhasorSimulation=off  OutputType=Complex  PSBequivalent=0
  Current Measurement2 : powerlib/Measurements/Current Measurement  PhasorSimulation=off  OutputType=Complex  PSBequivalent=0
  Grid : Subsystem
  Ground1 : powerlib/Elements/Ground  LConnTagsString=a
  Mux6 : Mux  Inputs=3
  Scope1 : Scope
  Series RLC Branch1 : powerlib/Elements/Series RLC Branch  LConnTagsString=__new0  RConnTagsString=__new0  BranchType=RL  Resistance=Rg_n2  Inductance=Lg_n2  SetiL0=off  InitialCurrent=0  Capacitance=0  Setx0=off  InitialVoltage=0  Measurements=None
  Series RLC Branch2 : powerlib/Elements/Series RLC Branch  LConnTagsString=__new0  RConnTagsString=__new0  BranchType=RL  Resistance=Rg_n1  Inductance=Lg_n1  SetiL0=off  InitialCurrent=0  Capacitance=0  Setx0=off  InitialVoltage=0  Measurements=None
  Series RLC Branch3 : powerlib/Elements/Series RLC Branch  LConnTagsString=__new0  RConnTagsString=__new0  BranchType=RL  Resistance=Rg_n1  Inductance=Lg_n1  SetiL0=off  InitialCurrent=0  Capacitance=0  Setx0=off  InitialVoltage=0  Measurements=None
  Series RLC Branch4 : powerlib/Elements/Series RLC Branch  LConnTagsString=__new0  RConnTagsString=__new0  BranchType=RL  Resistance=Rg_n2  Inductance=Lg_n2  SetiL0=off  InitialCurrent=0  Capacitance=0  Setx0=off  InitialVoltage=0  Measurements=None
  Series RLC Branch5 : powerlib/Elements/Series RLC Branch  LConnTagsString=__new0  RConnTagsString=__new0  BranchType=RL  Resistance=Rg_n2  Inductance=Lg_n2  SetiL0=off  InitialCurrent=0  Capacitance=0  Setx0=off  InitialVoltage=0  Measurements=None
  Series RLC Branch6 : powerlib/Elements/Series RLC Branch  LConnTagsString=__new0  RConnTagsString=__new0  BranchType=RL  Resistance=Rg_n1  Inductance=Lg_n1  SetiL0=off  InitialCurrent=0  Capacitance=0  Setx0=off  InitialVoltage=0  Measurements=None
  Series RLC Branch7 : powerlib/Elements/Series RLC Branch  Commented=on  LConnTagsString=__new0  RConnTagsString=__new0  BranchType=RL  Resistance=Rg_n1  Inductance=Lg_n1  SetiL0=off  InitialCurrent=0  Capacitance=0  Setx0=off  InitialVoltage=0  Measurements=None
  a : PMIOPort  Side=Right
  b : PMIOPort  Port=2  Side=Right
  c : PMIOPort  Port=3  Side=Right
  inabc : Outport
  wires:
  Mux6/1 -> inabc/1
  Grid/4(thetareal) -> Scope1/1
  Grid/1(vza) -> Controlled Voltage Source3/1
  Grid/2(vzb) -> Controlled Voltage Source4/1
  Grid/3(vzc) -> Controlled Voltage Source5/1
  Current Measurement10/1 -> Mux6/1
  Current Measurement1/1 -> Mux6/2
  Current Measurement2/1 -> Mux6/3
  connections:
  Current Measurement1/LConn1 -- b/RConn1
  Current Measurement2/LConn1 -- c/RConn1
  Current Measurement10/LConn1 -- a/RConn1
  Controlled Voltage Source4/LConn1 -- Ground1/LConn1 -- Controlled Voltage Source5/LConn1 -- Controlled Voltage Source3/LConn1
  Series RLC Branch3/RConn1 -- Series RLC Branch4/RConn1 -- Current Measurement2/RConn1
  Series RLC Branch3/LConn1 -- Series RLC Branch4/LConn1 -- Controlled Voltage Source5/RConn1
  Series RLC Branch2/RConn1 -- Current Measurement1/RConn1 -- Series RLC Branch1/RConn1
  Series RLC Branch2/LConn1 -- Series RLC Branch1/LConn1 -- Controlled Voltage Source4/RConn1
  Series RLC Branch6/LConn1 -- Controlled Voltage Source3/RConn1 -- Series RLC Branch5/LConn1
  Series RLC Branch5/RConn1 -- Current Measurement10/RConn1 -- Series RLC Branch6/RConn1

== system GFOL_nonlinear/P loop ==
  P_ref : Inport
  P_meas : Inport  Port=2
  u_qd : Inport  Port=3
  is_qd : Inport  Port=4
  Add2 : Sum
  Demux2 : Demux  Outputs=2
  Demux7 : Demux  Outputs=2
  Gain12 : Gain  Gain=3/2
  PID Controller : simulink/Continuous/PID Controller  Controller=PI  Form=Parallel  TimeDomain=Continuous-time  UseExternalTs=off  SampleTime=-1  IntegratorMethod=Forward Euler  FilterMethod=Forward Euler  ControllerParametersSource=internal  P=kp_P_n1  I=ki_P_n1  D=0  UseFilter=on  N=100  TunerSelectOption=Transfer Function Based (PID Tuner App)  InitialConditionSource=internal  InitialConditionForIntegrator=0  InitialConditionForFilter=0  DifferentiatorICPrevScaledInput=0  ExternalReset=none  TrackingMode=off  Kt=1  LimitOutput=off  UpperSaturationLimit=10*Ipeak_n1  LowerSaturationLimit=-10*Ipeak_n1  LinearizeAsGain=on  AntiWindupMode=clamping  Kb=1  POutMin=[]  POutMax=[]  IOutMin=[]  IOutMax=[]  DOutMin=[]  DOutMax=[]  NOutMin=[]  NOutMax=[]  SumOutMin=[]  SumOutMax=[]  SaturationOutMin=[]  SaturationOutMax=[]  PParamMin=[]  PParamMax=[]  IParamMin=[]  IParamMax=[]  DParamMin=[]  DParamMax=[]  NParamMin=[]  NParamMax=[]  KbParamMin=[]  KbParamMax=[]  KtParamMin=[]  KtParamMax=[]  KbOutMin=[]  KbOutMax=[]  KtOutMin=[]  KtOutMax=[]  IntegratorOutMin=[]  IntegratorOutMax=[]  FilterOutMin=[]  FilterOutMax=[]  SumI1OutMin=[]  SumI1OutMax=[]  SumI2OutMin=[]  SumI2OutMax=[]  SumI3OutMin=[]  SumI3OutMax=[]  SumI4OutMin=[]  SumI4OutMax=[]  SumDOutMin=[]  SumDOutMax=[]  DifferentiatorOutMin=[]  DifferentiatorOutMax=[]  FilterDiffOutCoefMin=[]  FilterDiffOutCoefMax=[]  ReciprocalOutMin=[]  ReciprocalOutMax=[]  SumDenOutMin=[]  SumDenOutMax=[]  SumNumOutMin=[]  SumNumOutMax=[]  DivideOutMin=[]  DivideOutMax=[]  UdiffTsProdOutMin=[]  UdiffTsProdOutMax=[]  NTsProdOutMin=[]  NTsProdOutMax=[]  UintegralTsProdOutMin=[]  UintegralTsProdOutMax=[]  UngainTsProdOutMin=[]  UngainTsProdOutMax=[]  IntegratorContinuousStateAttributes=''  IntegratorStateMustResolveToSignalObject=off  IntegratorRTWStateStorageClass=Auto  FilterContinuousStateAttributes=''  FilterStateMustResolveToSignalObject=off  FilterRTWStateStorageClass=Auto  ParallelPVariant=InternalParameters  IdealPVariant=Disabled  IVariant=InternalParameters  DVariant=Disabled  IntegratorVariant=Continuous  SatVariant=Disabled  AWVariant=Passthrough  PCopyVariant=Disabled  TRVariant=Disabled  FdbkBlocksVariant=Forward  IdealPFdbkVariant=Disabled  SatFdbkVariant=Disabled  DerivativeFilterVariant=Disabled  NVariant=Disabled  NCopyVariant=Disabled_SignalSpec  FilterICVariant=Disabled  IntegratorICVariant=InternalICs  ExternalResetVariant=Disabled  TRSumVariant=Passthrough  SumFdbkVariant=Disabled  SumVariant=Sum_PI  TsampFilterVariant=InternalTs  TsampNgainVariant=Passthrough  TsampIntegralVariant=Passthrough
  Product : Product
  Product1 : Product
  Scope3 : Scope
  Sum1 : Sum  Inputs=|+-
  is_q_ref : Outport
  P : Outport  Port=2
  wires:
  Sum1/1 -> Scope3/1, PID Controller/1
  PID Controller/1 -> is_q_ref/1
  P_meas/1 -> Sum1/2, P/1
  Product1/1 -> Add2/2
  Demux7/2 -> Product1/1
  Demux2/2 -> Product1/2
  Product/1 -> Add2/1
  Demux2/1 -> Product/2
  Demux7/1 -> Product/1
  Add2/1 -> Gain12/1
  u_qd/1 -> Demux7/1
  is_qd/1 -> Demux2/1
  P_ref/1 -> Sum1/1

== system GFOL_nonlinear/PLL ==
  u_abc : Inport
  Constant : Constant  Value=0
  Constant3 : Constant  Value=2*pi*f_n1
  Demux : Demux  Outputs=3
  Gain : Gain  Gain=1/(2*pi)
  Integrator : Integrator  WrappedStateUpperValue=2*pi  WrappedStateLowerValue=-2*pi
  PID Controller : simulink/Continuous/PID Controller  Controller=PI  Form=Parallel  TimeDomain=Continuous-time  UseExternalTs=off  SampleTime=-1  IntegratorMethod=Forward Euler  FilterMethod=Forward Euler  ControllerParametersSource=internal  P=kp_pll_n1  I=ki_pll_n1  D=0  UseFilter=on  N=100  TunerSelectOption=Transfer Function Based (PID Tuner App)  InitialConditionSource=internal  InitialConditionForIntegrator=0  InitialConditionForFilter=0  DifferentiatorICPrevScaledInput=0  ExternalReset=none  TrackingMode=off  Kt=1  LimitOutput=off  UpperSaturationLimit=0.5*2*pi*f_n1  LowerSaturationLimit=-0.5*2*pi*f_n1  LinearizeAsGain=on  AntiWindupMode=clamping  Kb=1  POutMin=[]  POutMax=[]  IOutMin=[]  IOutMax=[]  DOutMin=[]  DOutMax=[]  NOutMin=[]  NOutMax=[]  SumOutMin=[]  SumOutMax=[]  SaturationOutMin=[]  SaturationOutMax=[]  PParamMin=[]  PParamMax=[]  IParamMin=[]  IParamMax=[]  DParamMin=[]  DParamMax=[]  NParamMin=[]  NParamMax=[]  KbParamMin=[]  KbParamMax=[]  KtParamMin=[]  KtParamMax=[]  KbOutMin=[]  KbOutMax=[]  KtOutMin=[]  KtOutMax=[]  IntegratorOutMin=[]  IntegratorOutMax=[]  FilterOutMin=[]  FilterOutMax=[]  SumI1OutMin=[]  SumI1OutMax=[]  SumI2OutMin=[]  SumI2OutMax=[]  SumI3OutMin=[]  SumI3OutMax=[]  SumI4OutMin=[]  SumI4OutMax=[]  SumDOutMin=[]  SumDOutMax=[]  DifferentiatorOutMin=[]  DifferentiatorOutMax=[]  FilterDiffOutCoefMin=[]  FilterDiffOutCoefMax=[]  ReciprocalOutMin=[]  ReciprocalOutMax=[]  SumDenOutMin=[]  SumDenOutMax=[]  SumNumOutMin=[]  SumNumOutMax=[]  DivideOutMin=[]  DivideOutMax=[]  UdiffTsProdOutMin=[]  UdiffTsProdOutMax=[]  NTsProdOutMin=[]  NTsProdOutMax=[]  UintegralTsProdOutMin=[]  UintegralTsProdOutMax=[]  UngainTsProdOutMin=[]  UngainTsProdOutMax=[]  IntegratorContinuousStateAttributes=''  IntegratorStateMustResolveToSignalObject=off  IntegratorRTWStateStorageClass=Auto  FilterContinuousStateAttributes=''  FilterStateMustResolveToSignalObject=off  FilterRTWStateStorageClass=Auto  ParallelPVariant=InternalParameters  IdealPVariant=Disabled  IVariant=InternalParameters  DVariant=Disabled  IntegratorVariant=Continuous  SatVariant=Disabled  AWVariant=Passthrough  PCopyVariant=Disabled  TRVariant=Disabled  FdbkBlocksVariant=Forward  IdealPFdbkVariant=Disabled  SatFdbkVariant=Disabled  DerivativeFilterVariant=Disabled  NVariant=Disabled  NCopyVariant=Disabled_SignalSpec  FilterICVariant=Disabled  IntegratorICVariant=InternalICs  ExternalResetVariant=Disabled  TRSumVariant=Passthrough  SumFdbkVariant=Disabled  SumVariant=Sum_PI  TsampFilterVariant=InternalTs  TsampNgainVariant=Passthrough  TsampIntegralVariant=Passthrough
  ParkTransform : Subsystem  mask(Gerard){}
      mask help:
      | This block applies the park transfomation from a desired vector.
      | The input Xabc refers to the vector in the ABC frame, and the second input is the angle used in the transformation.
      | The output is the vector in the qd0 frame.
      mask Display:
      | port_label('output',1,'Xqd0')
      | port_label('input',1,'Xabc')
      | port_label('input',2,'angle')
  Scope1 : Scope
  Scope20 : Scope
  Sum : Sum  Inputs=|+-
  Sum1 : Sum  Inputs=|++
  Terminator8 : Terminator
  Vzq : Outport
  Vzd : Outport  Port=2
  angle : Outport  Port=3
  w_grid : Outport  Port=4
  wires:
  Constant3/1 -> Sum1/2
  Sum1/1 -> Gain/1, w_grid/1, Integrator/1
  Constant/1 -> Sum/1
  Integrator/1 -> ParkTransform/2(angle), angle/1
  Demux/3 -> Terminator8/1
  PID Controller/1 -> Sum1/1
  u_abc/1 -> ParkTransform/1(ABC vector)
  ParkTransform/1(Matrix) -> Demux/1
  Demux/1 -> Vzq/1
  Sum/1 -> PID Controller/1, Scope20/1
  Gain/1 -> Scope1/1
  Demux/2 -> Sum/2, Vzd/1

== system GFOL_nonlinear/PQ Calculation 1 ==
  u_qd : Inport
  ig_qd : Inport  Port=2
  Add1 : Sum  Inputs=-+
  Add2 : Sum
  Demux4 : Demux  Outputs=2
  Demux7 : Demux  Outputs=2
  Gain1 : Gain  Gain=3/2
  Gain12 : Gain  Gain=3/2
  Product{,1..3} (4 alike) : Product
  P : Outport
  Q : Outport  Port=2
  wires:
  Demux4/2 -> Product1/2, Product3/2
  Demux7/2 -> Product2/1, Product1/1
  Product/1 -> Add2/1
  Product1/1 -> Add2/2
  Add2/1 -> Gain12/1
  Demux7/1 -> Product3/1, Product/1
  Product2/1 -> Add1/1
  Demux4/1 -> Product2/2, Product/2
  Add1/1 -> Gain1/1
  Product3/1 -> Add1/2
  ig_qd/1 -> Demux4/1
  u_qd/1 -> Demux7/1
  Gain1/1 -> Q/1
  Gain12/1 -> P/1

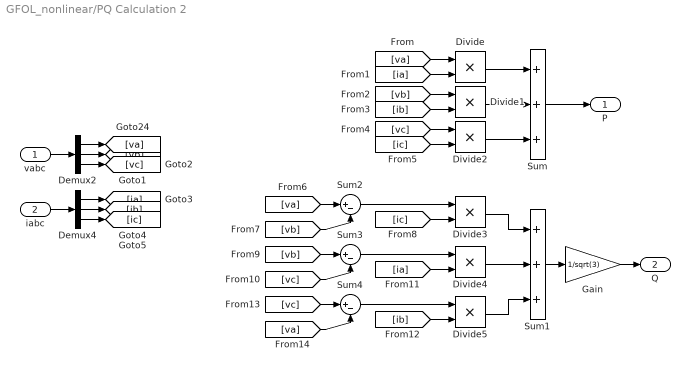
== system GFOL_nonlinear/PQ Calculation 2 ==
  vabc : Inport
  iabc : Inport  Port=2
  Demux2 : Demux  Outputs=3
  Demux4 : Demux  Outputs=3
  Divide{,1..5} (6 alike) : Product  Inputs=**
  Gain : Gain  Gain=1/sqrt(3)
  Sum : Sum  Inputs=+++
  Sum1 : Sum  Inputs=+++
  Sum2 : Sum  Inputs=|+-
  Sum3 : Sum  Inputs=|+-
  Sum4 : Sum  Inputs=|+-
  P : Outport
  Q : Outport  Port=2
  wires:
  vabc/1 -> Demux2/1
  iabc/1 -> Demux4/1
  Demux2/1 -> [va]
  Demux2/2 -> [vb]
  Demux2/3 -> [vc]
  Demux4/1 -> [ia]
  Demux4/2 -> [ib]
  Demux4/3 -> [ic]
  Divide/1 -> Sum/1
  [ia] -> Divide/2
  [va] -> Divide/1
  Divide1/1 -> Sum/2
  [vb] -> Divide1/1
  [ib] -> Divide1/2
  Divide2/1 -> Sum/3
  [vc] -> Divide2/1
  [ic] -> Divide2/2
  Sum/1 -> P/1
  Sum1/1 -> Gain/1
  [ib] -> Divide5/2
  Sum4/1 -> Divide5/1
  Divide5/1 -> Sum1/3
  [ia] -> Divide4/2
  Sum3/1 -> Divide4/1
  Divide4/1 -> Sum1/2
  Sum2/1 -> Divide3/1
  [ic] -> Divide3/2
  Divide3/1 -> Sum1/1
  [va] -> Sum2/1
  [vb] -> Sum2/2
  [vb] -> Sum3/1
  [vc] -> Sum3/2
  [vc] -> Sum4/1
  [va] -> Sum4/2
  Gain/1 -> Q/1

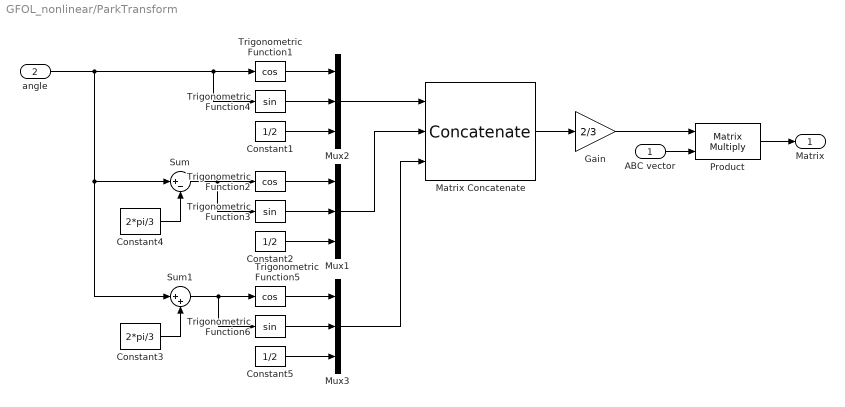
== system GFOL_nonlinear/ParkTransform ==
  ABC vector : Inport
  angle : Inport  Port=2
  Constant1 : Constant  Value=1/2
  Constant2 : Constant  Value=1/2
  Constant3 : Constant  Value=2*pi/3
  Constant4 : Constant  Value=2*pi/3
  Constant5 : Constant  Value=1/2
  Gain : Gain  Gain=2/3
  Matrix Concatenate : Concatenate  NumInputs=3  Mode=Multidimensional array  ConcatenateDimension=2
  Mux1 : Mux  Inputs=3
  Mux2 : Mux  Inputs=3
  Mux3 : Mux  Inputs=3
  Product : Product  Multiplication=Matrix(*)  RndMeth=Zero
  Sum : Sum  Inputs=|+-
  Sum1 : Sum  Inputs=|++
  Trigonometric Function1 : Trigonometry  Operator=cos
  Trigonometric Function2 : Trigonometry  Operator=cos
  Trigonometric Function3 : Trigonometry
  Trigonometric Function4 : Trigonometry
  Trigonometric Function5 : Trigonometry  Operator=cos
  Trigonometric Function6 : Trigonometry
  Matrix : Outport
  wires:
  Matrix Concatenate/1 -> Gain/1
  ABC vector/1 -> Product/2
  Product/1 -> Matrix/1
  Gain/1 -> Product/1
  Constant4/1 -> Sum/2
  Constant3/1 -> Sum1/2
  angle/1 -> Trigonometric Function4/1, Trigonometric Function1/1, Sum1/1, Sum/1
  Trigonometric Function3/1 -> Mux1/2
  Trigonometric Function2/1 -> Mux1/1
  Constant2/1 -> Mux1/3
  Sum/1 -> Trigonometric Function3/1, Trigonometric Function2/1
  Trigonometric Function4/1 -> Mux2/2
  Trigonometric Function1/1 -> Mux2/1
  Constant1/1 -> Mux2/3
  Trigonometric Function6/1 -> Mux3/2
  Trigonometric Function5/1 -> Mux3/1
  Constant5/1 -> Mux3/3
  Sum1/1 -> Trigonometric Function6/1, Trigonometric Function5/1
  Mux1/1 -> Matrix Concatenate/2
  Mux2/1 -> Matrix Concatenate/1
  Mux3/1 -> Matrix Concatenate/3

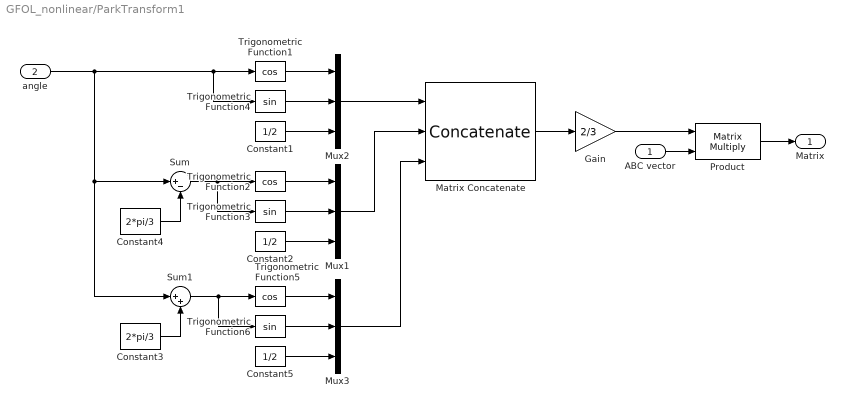
== system GFOL_nonlinear/ParkTransform1 ==
  ABC vector : Inport
  angle : Inport  Port=2
  Constant1 : Constant  Value=1/2
  Constant2 : Constant  Value=1/2
  Constant3 : Constant  Value=2*pi/3
  Constant4 : Constant  Value=2*pi/3
  Constant5 : Constant  Value=1/2
  Gain : Gain  Gain=2/3
  Matrix Concatenate : Concatenate  NumInputs=3  Mode=Multidimensional array  ConcatenateDimension=2
  Mux1 : Mux  Inputs=3
  Mux2 : Mux  Inputs=3
  Mux3 : Mux  Inputs=3
  Product : Product  Multiplication=Matrix(*)  RndMeth=Zero
  Sum : Sum  Inputs=|+-
  Sum1 : Sum  Inputs=|++
  Trigonometric Function1 : Trigonometry  Operator=cos
  Trigonometric Function2 : Trigonometry  Operator=cos
  Trigonometric Function3 : Trigonometry
  Trigonometric Function4 : Trigonometry
  Trigonometric Function5 : Trigonometry  Operator=cos
  Trigonometric Function6 : Trigonometry
  Matrix : Outport
  wires:
  Mux3/1 -> Matrix Concatenate/3
  Mux2/1 -> Matrix Concatenate/1
  Mux1/1 -> Matrix Concatenate/2
  Sum1/1 -> Trigonometric Function5/1, Trigonometric Function6/1
  Constant5/1 -> Mux3/3
  Trigonometric Function5/1 -> Mux3/1
  Trigonometric Function6/1 -> Mux3/2
  Constant1/1 -> Mux2/3
  Trigonometric Function1/1 -> Mux2/1
  Trigonometric Function4/1 -> Mux2/2
  Sum/1 -> Trigonometric Function2/1, Trigonometric Function3/1
  Constant2/1 -> Mux1/3
  Trigonometric Function2/1 -> Mux1/1
  Trigonometric Function3/1 -> Mux1/2
  angle/1 -> Sum/1, Sum1/1, Trigonometric Function1/1, Trigonometric Function4/1
  Constant3/1 -> Sum1/2
  Constant4/1 -> Sum/2
  Gain/1 -> Product/1
  Product/1 -> Matrix/1
  ABC vector/1 -> Product/2
  Matrix Concatenate/1 -> Gain/1

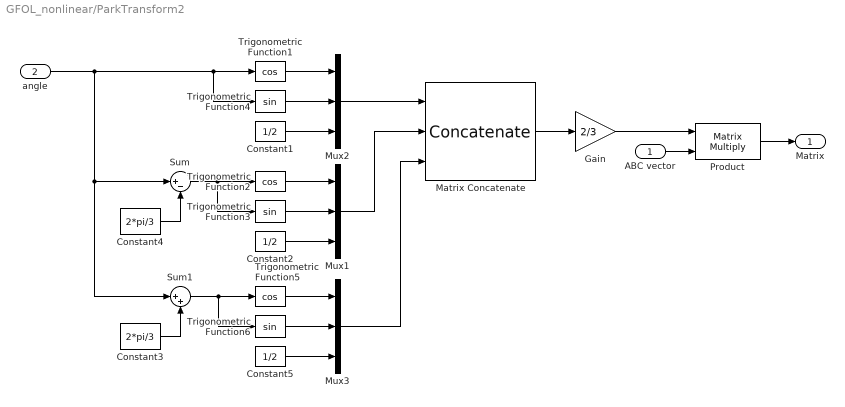
== system GFOL_nonlinear/ParkTransform2 ==
  ABC vector : Inport
  angle : Inport  Port=2
  Constant1 : Constant  Value=1/2
  Constant2 : Constant  Value=1/2
  Constant3 : Constant  Value=2*pi/3
  Constant4 : Constant  Value=2*pi/3
  Constant5 : Constant  Value=1/2
  Gain : Gain  Gain=2/3
  Matrix Concatenate : Concatenate  NumInputs=3  Mode=Multidimensional array  ConcatenateDimension=2
  Mux1 : Mux  Inputs=3
  Mux2 : Mux  Inputs=3
  Mux3 : Mux  Inputs=3
  Product : Product  Multiplication=Matrix(*)  RndMeth=Zero
  Sum : Sum  Inputs=|+-
  Sum1 : Sum  Inputs=|++
  Trigonometric Function1 : Trigonometry  Operator=cos
  Trigonometric Function2 : Trigonometry  Operator=cos
  Trigonometric Function3 : Trigonometry
  Trigonometric Function4 : Trigonometry
  Trigonometric Function5 : Trigonometry  Operator=cos
  Trigonometric Function6 : Trigonometry
  Matrix : Outport
  wires:
  Mux3/1 -> Matrix Concatenate/3
  Mux2/1 -> Matrix Concatenate/1
  Mux1/1 -> Matrix Concatenate/2
  Sum1/1 -> Trigonometric Function5/1, Trigonometric Function6/1
  Constant5/1 -> Mux3/3
  Trigonometric Function5/1 -> Mux3/1
  Trigonometric Function6/1 -> Mux3/2
  Constant1/1 -> Mux2/3
  Trigonometric Function1/1 -> Mux2/1
  Trigonometric Function4/1 -> Mux2/2
  Sum/1 -> Trigonometric Function2/1, Trigonometric Function3/1
  Constant2/1 -> Mux1/3
  Trigonometric Function2/1 -> Mux1/1
  Trigonometric Function3/1 -> Mux1/2
  angle/1 -> Sum/1, Sum1/1, Trigonometric Function1/1, Trigonometric Function4/1
  Constant3/1 -> Sum1/2
  Constant4/1 -> Sum/2
  Gain/1 -> Product/1
  Product/1 -> Matrix/1
  ABC vector/1 -> Product/2
  Matrix Concatenate/1 -> Gain/1

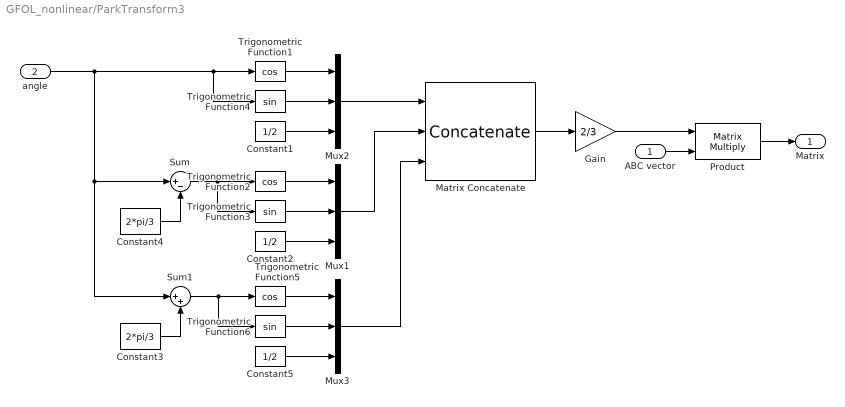
== system GFOL_nonlinear/ParkTransform3 ==
  ABC vector : Inport
  angle : Inport  Port=2
  Constant1 : Constant  Value=1/2
  Constant2 : Constant  Value=1/2
  Constant3 : Constant  Value=2*pi/3
  Constant4 : Constant  Value=2*pi/3
  Constant5 : Constant  Value=1/2
  Gain : Gain  Gain=2/3
  Matrix Concatenate : Concatenate  NumInputs=3  Mode=Multidimensional array  ConcatenateDimension=2
  Mux1 : Mux  Inputs=3
  Mux2 : Mux  Inputs=3
  Mux3 : Mux  Inputs=3
  Product : Product  Multiplication=Matrix(*)  RndMeth=Zero
  Sum : Sum  Inputs=|+-
  Sum1 : Sum  Inputs=|++
  Trigonometric Function1 : Trigonometry  Operator=cos
  Trigonometric Function2 : Trigonometry  Operator=cos
  Trigonometric Function3 : Trigonometry
  Trigonometric Function4 : Trigonometry
  Trigonometric Function5 : Trigonometry  Operator=cos
  Trigonometric Function6 : Trigonometry
  Matrix : Outport
  wires:
  Matrix Concatenate/1 -> Gain/1
  ABC vector/1 -> Product/2
  Product/1 -> Matrix/1
  Gain/1 -> Product/1
  Constant4/1 -> Sum/2
  Constant3/1 -> Sum1/2
  angle/1 -> Trigonometric Function4/1, Trigonometric Function1/1, Sum1/1, Sum/1
  Trigonometric Function3/1 -> Mux1/2
  Trigonometric Function2/1 -> Mux1/1
  Constant2/1 -> Mux1/3
  Sum/1 -> Trigonometric Function3/1, Trigonometric Function2/1
  Trigonometric Function4/1 -> Mux2/2
  Trigonometric Function1/1 -> Mux2/1
  Constant1/1 -> Mux2/3
  Trigonometric Function6/1 -> Mux3/2
  Trigonometric Function5/1 -> Mux3/1
  Constant5/1 -> Mux3/3
  Sum1/1 -> Trigonometric Function6/1, Trigonometric Function5/1
  Mux1/1 -> Matrix Concatenate/2
  Mux2/1 -> Matrix Concatenate/1
  Mux3/1 -> Matrix Concatenate/3

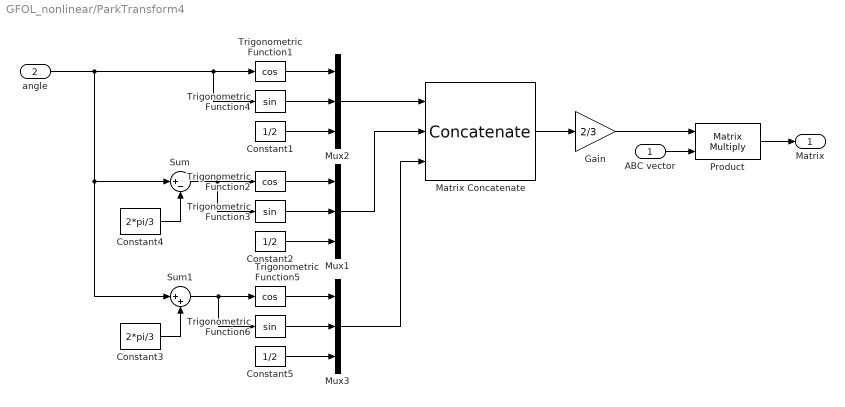
== system GFOL_nonlinear/ParkTransform4 ==
  ABC vector : Inport
  angle : Inport  Port=2
  Constant1 : Constant  Value=1/2
  Constant2 : Constant  Value=1/2
  Constant3 : Constant  Value=2*pi/3
  Constant4 : Constant  Value=2*pi/3
  Constant5 : Constant  Value=1/2
  Gain : Gain  Gain=2/3
  Matrix Concatenate : Concatenate  NumInputs=3  Mode=Multidimensional array  ConcatenateDimension=2
  Mux1 : Mux  Inputs=3
  Mux2 : Mux  Inputs=3
  Mux3 : Mux  Inputs=3
  Product : Product  Multiplication=Matrix(*)  RndMeth=Zero
  Sum : Sum  Inputs=|+-
  Sum1 : Sum  Inputs=|++
  Trigonometric Function1 : Trigonometry  Operator=cos
  Trigonometric Function2 : Trigonometry  Operator=cos
  Trigonometric Function3 : Trigonometry
  Trigonometric Function4 : Trigonometry
  Trigonometric Function5 : Trigonometry  Operator=cos
  Trigonometric Function6 : Trigonometry
  Matrix : Outport
  wires:
  Matrix Concatenate/1 -> Gain/1
  ABC vector/1 -> Product/2
  Product/1 -> Matrix/1
  Gain/1 -> Product/1
  Constant4/1 -> Sum/2
  Constant3/1 -> Sum1/2
  angle/1 -> Trigonometric Function4/1, Trigonometric Function1/1, Sum1/1, Sum/1
  Trigonometric Function3/1 -> Mux1/2
  Trigonometric Function2/1 -> Mux1/1
  Constant2/1 -> Mux1/3
  Sum/1 -> Trigonometric Function3/1, Trigonometric Function2/1
  Trigonometric Function4/1 -> Mux2/2
  Trigonometric Function1/1 -> Mux2/1
  Constant1/1 -> Mux2/3
  Trigonometric Function6/1 -> Mux3/2
  Trigonometric Function5/1 -> Mux3/1
  Constant5/1 -> Mux3/3
  Sum1/1 -> Trigonometric Function6/1, Trigonometric Function5/1
  Mux1/1 -> Matrix Concatenate/2
  Mux2/1 -> Matrix Concatenate/1
  Mux3/1 -> Matrix Concatenate/3

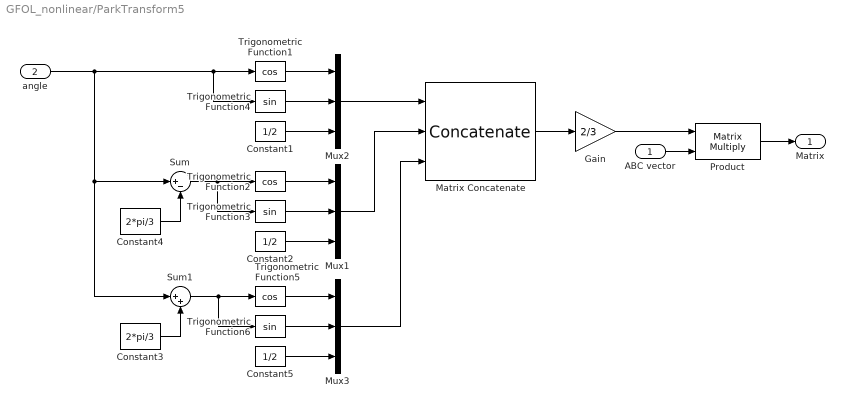
== system GFOL_nonlinear/ParkTransform5 ==
  ABC vector : Inport
  angle : Inport  Port=2
  Constant1 : Constant  Value=1/2
  Constant2 : Constant  Value=1/2
  Constant3 : Constant  Value=2*pi/3
  Constant4 : Constant  Value=2*pi/3
  Constant5 : Constant  Value=1/2
  Gain : Gain  Gain=2/3
  Matrix Concatenate : Concatenate  NumInputs=3  Mode=Multidimensional array  ConcatenateDimension=2
  Mux1 : Mux  Inputs=3
  Mux2 : Mux  Inputs=3
  Mux3 : Mux  Inputs=3
  Product : Product  Multiplication=Matrix(*)  RndMeth=Zero
  Sum : Sum  Inputs=|+-
  Sum1 : Sum  Inputs=|++
  Trigonometric Function1 : Trigonometry  Operator=cos
  Trigonometric Function2 : Trigonometry  Operator=cos
  Trigonometric Function3 : Trigonometry
  Trigonometric Function4 : Trigonometry
  Trigonometric Function5 : Trigonometry  Operator=cos
  Trigonometric Function6 : Trigonometry
  Matrix : Outport
  wires:
  Matrix Concatenate/1 -> Gain/1
  ABC vector/1 -> Product/2
  Product/1 -> Matrix/1
  Gain/1 -> Product/1
  Constant4/1 -> Sum/2
  Constant3/1 -> Sum1/2
  angle/1 -> Trigonometric Function4/1, Trigonometric Function1/1, Sum1/1, Sum/1
  Trigonometric Function3/1 -> Mux1/2
  Trigonometric Function2/1 -> Mux1/1
  Constant2/1 -> Mux1/3
  Sum/1 -> Trigonometric Function3/1, Trigonometric Function2/1
  Trigonometric Function4/1 -> Mux2/2
  Trigonometric Function1/1 -> Mux2/1
  Constant1/1 -> Mux2/3
  Trigonometric Function6/1 -> Mux3/2
  Trigonometric Function5/1 -> Mux3/1
  Constant5/1 -> Mux3/3
  Sum1/1 -> Trigonometric Function6/1, Trigonometric Function5/1
  Mux1/1 -> Matrix Concatenate/2
  Mux2/1 -> Matrix Concatenate/1
  Mux3/1 -> Matrix Concatenate/3
